simulink model "qless_forgetting_factor_16x16"  (R2021a)
settings: Solver=FixedStepDiscrete  StartTime=0.0  StopTime=stoptime*inf  RelTol=1e-3
InitFcn:
  | qless_init_16chan_fi
undefined symbols (not defined in the file): fc, numArrayElements, physconst, srcAngles, sv, Ts
libraries: hdlsllib x137, commfilt2 x4, commrfcorlib x3, commsync2 x3, commrflib2 x2, commrandsrc3 x2, phasedtxrxlib x2, commdigbbndcpm2 x1, simulink x1, embreciprocals x1, commdigbbndpm3 x1
(part 15 of 22)

== matlab function qless_forgetting_factor_16x16/MVDR_QLess_HDL/Complex Partial-Systolic Matrix Solve Using Q-less QR Decomposition with Forgetting Factor Manually Tiled n=16/Complex Partial-Systolic Q-less QR with Forgetting Factor/Complex Partial-Systolic Q-less QR with Forgetting Factor Manually tiled/Complex Partial-Systolic Q-less QR Decomposition with Forgetting Factor Section Constant pivot2/Partial-Systolic Q-less QR with Forgetting Factor Memory Controller/MATLAB Function ==
  data: xIn input; xOut output; aIn input; validIn input size=1; validRowRotationInput input size=1; restart input size=1; yOut output; processRowRotations output size=1; validOut output size=1; ready output size=1; n parameter size=1
function [...
        xOut,...
        yOut,...
        processRowRotations,...
        validOut,...
        ready...
        ] = ...
        partialSystolicQlessQRMemoryControllerForgettingFactorMATLAB(...
        xIn,...
        aIn,...
        validIn,...
        validRowRotationInput,...
        restart, ...
        n)
    
    % Persistent states
    persistent mState
    persistent mRow
    persistent mR
    
    if isempty(mState)
        mState = uint8(0);
        mRow = uint16(1);
        mR = zeros(1,n,'like',aIn);
    end
    
    [...
        xOut,...
        yOut,...
        processRowRotations,...
        validOut,...
        ready,...
        mState,...
        mRow,...
        mR...
        ] = ...
        partialSystolicQlessQRMemoryControllerForgettingFactor(...
        xIn,...
        aIn,...
        validIn,...
        validRowRotationInput,...
        restart, ...
        n,...
        mState,...
        mRow,...
        mR);
end

function [...
        xOut,...
        yOut,...
        processRowRotations,...
        validOut,...
        ready,...
        mState,...
        mRowIndex,...
        mRow...
        ] = ...
        partialSystolicQlessQRMemoryControllerForgettingFactor(...
        xIn,...
        aIn,...
        validIn,...
        validRowRotationInput,...
        restart, ...
        n,...
        mState,...
        mRowIndex,...
        mRow)
    %partialSystolicQlessQRMemoryControllerForgettingFactor
    
    % Copyright 2020 The MathWorks, Inc.
    %#codegen
    
    % State names
    NEWMATRIX = uint8(0);
    GETROW = uint8(1);
    PROCESSPIVOT = uint8(2);
    OUTPUTROW = uint8(3);
    
    % Get states
    state = mState;
    row = mRowIndex;
    
    if restart
        state = NEWMATRIX;
    end
    
    % Default outputs.  States change them as needed.
    xOut = mRow;
    yOut = aIn;
    processRowRotations = false;
    validOut = false;
    ready = false;
    
    switch state
        case NEWMATRIX
            mRow(:) = 0;
            mRowIndex(:) = 1;
            mState(:) = GETROW;
            ready(:) = true;
        case GETROW
            if  validIn
                processRowRotations = true;
                mRowIndex(:) = row + 1;
                mState(:) = PROCESSPIVOT;
            else
                ready = true;
            end
        case PROCESSPIVOT
            if validRowRotationInput
                mRow(:) = xIn;
                if row > n
                    mState(:) = OUTPUTROW;
                else
                    mState(:) = GETROW;
                end
            end
        case OUTPUTROW
            validOut = true;
            mState(:) = GETROW;
    end
end

== matlab function qless_forgetting_factor_16x16/MVDR_QLess_HDL/Complex Partial-Systolic Matrix Solve Using Q-less QR Decomposition with Forgetting Factor Manually Tiled n=16/Complex Partial-Systolic Q-less QR with Forgetting Factor/Complex Partial-Systolic Q-less QR with Forgetting Factor Manually tiled/Complex Partial-Systolic Q-less QR Decomposition with Forgetting Factor Section Constant pivot1/Complex Partial-Systolic Q-less QR Row Rotations/Q-less QR 2nd and 3rd Quadrant Compensation ==
  settings: fimath=hdlfimath
  data: x input size=[1,n]; y input size=[1,n]; xOut output size=[1,n]; yOut output size=[1,n]; pivot parameter size=1
function [xOut, yOut] = quadrantCompensation(x, y, pivot)
    %quadrantCompensation Quadrant adjustment by reflection through the origin.
    %   [XOUT, YOUT, UOUT, VOUT] = QUADRANT_COMPENSATION(X,Y,U,V,PIVOT)
    %   reflects the points (x,y) and (u,v) through the origin if (x,y)
    %   lies in the 3rd or 4th quadrant. This brings the points into the
    %   1st and 2nd quadrants for CORDIC algorithms.
    
    %   Copyright 2018 The MathWorks, Inc.
    %#codegen

   if real(x(pivot))<0
        % Compensation for 3rd and 4th quadrants
        xOut = -x;
        yOut = -y;
    else
        xOut = x;
        yOut = y;
    end


end

== matlab function qless_forgetting_factor_16x16/MVDR_QLess_HDL/Complex Partial-Systolic Matrix Solve Using Q-less QR Decomposition with Forgetting Factor Manually Tiled n=16/Complex Partial-Systolic Q-less QR with Forgetting Factor/Complex Partial-Systolic Q-less QR with Forgetting Factor Manually tiled/Complex Partial-Systolic Q-less QR Decomposition with Forgetting Factor Section Constant pivot3/Complex Partial-Systolic Q-less QR Row Rotations/Complex Partial-Systolic Q-less QR CORDIC Row Rotation/CORDIC QR Kernel ==
  settings: fimath=hdlfimath
  data: xIn input; yIn input; validIn input; restart input; xOut output size=[1 n]; yOut output size=[1 n]; n parameter; validOut output boolean; ready output; pivot parameter size=1
function [xOut, yOut, validOut, ready] = cordic_qr_row_rotation(...
                                                xIn, yIn,...
                                                validIn,...
                                                restart,...
                                                n, pivot)... 
    %CORDIC_QR_ROW_ROTATION performs one CORDIC Givens rotation
    % [XOUT, YOUT] = CORDIC_QR_ROW_ROTATION(...
    %                                       XREG,YREG,...
    %                                       XIN,YIN,...
    %                                       pivot,...
    %                                       STILLITERATING, ITERATION)
    % performs one iteration of the CORDIC Givens rotation according to
    % the formula below.
    %
    % if real(y(column)) < 0
    %       xOut = x - y/2^iteration
    %       yOut = y + x/2^iteration
    %   else
    %       xOut = x + y/2^iteration
    %       yOut = y - x/2^iteration
    % end
    %
    % The values for X, Y, are taken from XIN, YIN, on the first iteration, 
    % and XREG, YREG on succeeding iterations.
    
    %   Copyright 2018 The MathWorks, Inc.
    
    %#codegen
    
    % Initialize variables to set datatypes
    
    persistent xReg yReg count readyReg
    
    
    
    fixed.emblib.internal.cordicRowRotations.checkValidDatatypes(xIn, yIn,'x','y', 'cordic_qr_row_rotation');
    T = fixed.emblib.internal.cordicRowRotations.getTypesTable(xIn,xIn);
    maxNIters = coder.const(fixed.emblib.internal.cordicRowRotations.getMaxNIters(xIn));
    
    if isempty(xReg)
       xReg = zeros(1,n,'like',T.x);
       yReg = zeros(1,n,'like',T.y);
       count = cast(0,'like',T.count);
       readyReg = true;
    end
    
    if validIn
        iteration = cast(0,'like',count);
        x = cast(xIn,'like',T.x);
        y = cast(yIn,'like',T.y);
    else
        iteration = count;
        x = xReg;
        y = yReg;
    end
    
    [xNext, yNext] = cordicQlessQRRowRotation(x, y, iteration, pivot, T);
    incrCounter =  (validIn && readyReg) || (iteration > 0 && iteration < maxNIters);
    if restart || ~incrCounter
        iterationNext = cast(0,'like',T.count);
    else
        iterationNext = cast(iteration + 1,'like',T.count);
    end
    
    if restart || (iteration == maxNIters - 1)
        readyNext = true;
    elseif validIn && ~readyReg
        readyNext = false;
    else
        readyNext = readyReg;
    end
        
        
    % Set the output
    xOut = xNext;
    yOut = yNext;
    if iteration == maxNIters - 1
        validOut = true;
        % Set the registers to zero to prevent overflows being reported on
        % CORDIC iterations over invalid data.
        xReg(:) = 0;
        yReg(:) = 0;
    else
        validOut = false;
        % Still iterating, so update the registers with next values.    
        xReg(:) = xNext;
        yReg(:) = yNext;
    end
    ready = readyNext;
    % Update the registers
    count(:) = iterationNext;
    readyReg(:) = readyNext;
    
end

function [xOut, yOut] = cordicQlessQRRowRotation(x, y,...
        iteration, pivot, T)
%cordicQlessQRRowRotation One iteration of the Q-less QR CORDIC kernel
%   [XOUT, YOUT] = cordicQlessQRRowRotation(X,Y,...
%                                      ITERATION, PIVOT, T)
%   performs a single CORDIC Givens rotation according to the
%   formula below
%
%   if real(y(pivot)) < 0
%       xOut = x - y/2^iteration
%       yOut = y + x/2^iteration
%   else
%       xOut = x + y/2^iteration
%       yOut = y - x/2^iteration
%   end

    coder.inline('always');
    
    % Initialize output variables
    xOut = cast(x,'like',T.x);
    yOut = cast(y,'like',T.y);
    % Right shift the inputs for CORDIC rotations.
    x1 = zeros(size(x),'like',x);
    y1 = zeros(size(y),'like',y);
    coder.unroll
    for k = pivot:length(x)
        x1(k) = bitsra(x(k), iteration);
        y1(k) = bitsra(y(k), iteration);
    end
    if real(y(pivot)) < 0
        % Counter-clockwise rotation
        coder.unroll
        for k = pivot:length(x)
            xOut(k) = x(k) - y1(k);
            yOut(k) = y(k) + x1(k);
        end
    else
        % Clockwise rotation
        coder.unroll
        for k = pivot:length(x)
            xOut(k) = x(k) + y1(k);
            yOut(k) = y(k) - x1(k);
        end
    end
end

== matlab function qless_forgetting_factor_16x16/MVDR_QLess_HDL/Complex Partial-Systolic Matrix Solve Using Q-less QR Decomposition with Forgetting Factor Manually Tiled n=16/Complex Partial-Systolic Q-less QR with Forgetting Factor/Complex Partial-Systolic Q-less QR with Forgetting Factor Manually tiled/Complex Partial-Systolic Q-less QR Decomposition with Forgetting Factor Section Constant pivot3/Complex Partial-Systolic Q-less QR Row Rotations/Inverse CORDIC Gain1/MATLAB Function ==
  data: u input; y output
function y = inverseCORDICGain(u)
    %inverseCORDICGain Multiply by the inverse of the CORDIC gain constant
    %   Y = inverseCORDICGain(U) multiplies input U by the inverse CORDIC
    %   gain constant.  The data type of output Y is the same as the data
    %   type of input U.  This data type will never overflow because the
    %   inverse CORDIC gain constant quickly converges to around 0.60725 as
    %   a function of the word length of the input.
    F = fixed.fimathLike(u);
    [~, Kn] = fixed.cordicConstants(u);
    y = setfimath(u,F) * Kn;
end

== matlab function qless_forgetting_factor_16x16/MVDR_QLess_HDL/Complex Partial-Systolic Matrix Solve Using Q-less QR Decomposition with Forgetting Factor Manually Tiled n=16/Complex Partial-Systolic Q-less QR with Forgetting Factor/Complex Partial-Systolic Q-less QR with Forgetting Factor Manually tiled/Complex Partial-Systolic Q-less QR Decomposition with Forgetting Factor Section Constant pivot3/Complex Partial-Systolic Q-less QR Row Rotations/Inverse CORDIC Gain4/MATLAB Function ==
  data: u input; y output
function y = inverseCORDICGain(u)
    %inverseCORDICGain Multiply by the inverse of the CORDIC gain constant
    %   Y = inverseCORDICGain(U) multiplies input U by the inverse CORDIC
    %   gain constant.  The data type of output Y is the same as the data
    %   type of input U.  This data type will never overflow because the
    %   inverse CORDIC gain constant quickly converges to around 0.60725 as
    %   a function of the word length of the input.
    F = fixed.fimathLike(u);
    [~, Kn] = fixed.cordicConstants(u);
    y = setfimath(u,F) * Kn;
end

== matlab function qless_forgetting_factor_16x16/MVDR_QLess_HDL/Complex Partial-Systolic Matrix Solve Using Q-less QR Decomposition with Forgetting Factor Manually Tiled n=16/Complex Partial-Systolic Q-less QR with Forgetting Factor/Complex Partial-Systolic Q-less QR with Forgetting Factor Manually tiled/Complex Partial-Systolic Q-less QR Decomposition with Forgetting Factor Section Constant pivot3/Complex Partial-Systolic Q-less QR Row Rotations/Q-less QR 2nd and 3rd Quadrant Compensation ==
  settings: fimath=hdlfimath
  data: x input size=[1,n]; y input size=[1,n]; xOut output size=[1,n]; yOut output size=[1,n]; pivot parameter size=1
function [xOut, yOut] = quadrantCompensation(x, y, pivot)
    %quadrantCompensation Quadrant adjustment by reflection through the origin.
    %   [XOUT, YOUT, UOUT, VOUT] = QUADRANT_COMPENSATION(X,Y,U,V,PIVOT)
    %   reflects the points (x,y) and (u,v) through the origin if (x,y)
    %   lies in the 3rd or 4th quadrant. This brings the points into the
    %   1st and 2nd quadrants for CORDIC algorithms.
    
    %   Copyright 2018 The MathWorks, Inc.
    %#codegen

   if real(x(pivot))<0
        % Compensation for 3rd and 4th quadrants
        xOut = -x;
        yOut = -y;
    else
        xOut = x;
        yOut = y;
    end


end

== matlab function qless_forgetting_factor_16x16/MVDR_QLess_HDL/Complex Partial-Systolic Matrix Solve Using Q-less QR Decomposition with Forgetting Factor Manually Tiled n=16/Complex Partial-Systolic Q-less QR with Forgetting Factor/Complex Partial-Systolic Q-less QR with Forgetting Factor Manually tiled/Complex Partial-Systolic Q-less QR Decomposition with Forgetting Factor Section Constant pivot3/Complex Partial-Systolic Q-less QR Row Rotations/Q-less QR Rotate First Element To Real1/Q-less QR Real Row Rotations/Inverse CORDIC Gain/MATLAB Function ==
  data: u input; y output
function y = inverseCORDICGain(u)
    %inverseCORDICGain Multiply by the inverse of the CORDIC gain constant
    %   Y = inverseCORDICGain(U) multiplies input U by the inverse CORDIC
    %   gain constant.  The data type of output Y is the same as the data
    %   type of input U.  This data type will never overflow because the
    %   inverse CORDIC gain constant quickly converges to around 0.60725 as
    %   a function of the word length of the input.
    F = fixed.fimathLike(u);
    [~, Kn] = fixed.cordicConstants(u);
    y = setfimath(u,F) * Kn;
end

== matlab function qless_forgetting_factor_16x16/MVDR_QLess_HDL/Complex Partial-Systolic Matrix Solve Using Q-less QR Decomposition with Forgetting Factor Manually Tiled n=16/Complex Partial-Systolic Q-less QR with Forgetting Factor/Complex Partial-Systolic Q-less QR with Forgetting Factor Manually tiled/Complex Partial-Systolic Q-less QR Decomposition with Forgetting Factor Section Constant pivot3/Complex Partial-Systolic Q-less QR Row Rotations/Q-less QR Rotate First Element To Real1/Q-less QR Real Row Rotations/Inverse CORDIC Gain1/MATLAB Function ==
  data: u input; y output
function y = inverseCORDICGain(u)
    %inverseCORDICGain Multiply by the inverse of the CORDIC gain constant
    %   Y = inverseCORDICGain(U) multiplies input U by the inverse CORDIC
    %   gain constant.  The data type of output Y is the same as the data
    %   type of input U.  This data type will never overflow because the
    %   inverse CORDIC gain constant quickly converges to around 0.60725 as
    %   a function of the word length of the input.
    F = fixed.fimathLike(u);
    [~, Kn] = fixed.cordicConstants(u);
    y = setfimath(u,F) * Kn;
end

== matlab function qless_forgetting_factor_16x16/MVDR_QLess_HDL/Complex Partial-Systolic Matrix Solve Using Q-less QR Decomposition with Forgetting Factor Manually Tiled n=16/Complex Partial-Systolic Q-less QR with Forgetting Factor/Complex Partial-Systolic Q-less QR with Forgetting Factor Manually tiled/Complex Partial-Systolic Q-less QR Decomposition with Forgetting Factor Section Constant pivot3/Complex Partial-Systolic Q-less QR Row Rotations/Q-less QR Rotate First Element To Real1/Q-less QR Real Row Rotations/Q-less QR Real Indexed CORDIC Row Rotation/CORDIC QR Kernel ==
  settings: fimath=hdlfimath
  data: xIn input size=n; yIn input size=n; validIn input; restart input; xOut output size=n; yOut output size=n; n parameter; validOut output boolean; ready output; pivot parameter size=1
function [xOut, yOut, validOut, ready] = cordic_qr_row_rotation(...
                                                xIn, yIn,...
                                                validIn,...
                                                restart,...
                                                n, pivot)... 
    %CORDIC_QR_ROW_ROTATION performs one CORDIC Givens rotation
    % [XOUT, YOUT] = CORDIC_QR_ROW_ROTATION(...
    %                                       XREG,YREG,...
    %                                       XIN,YIN,...
    %                                       PIVOT,...
    %                                       STILLITERATING, ITERATION)
    % performs one iteration of the CORDIC Givens rotation according to
    % the formula below.
    %
    % if real(y(column)) < 0
    %       xOut = x - y/2^iteration
    %       yOut = y + x/2^iteration
    %   else
    %       xOut = x + y/2^iteration
    %       yOut = y - x/2^iteration
    % end
    %
    % The values for X, Y, are taken from XIN, YIN, on the first iteration, 
    % and XREG, YREG on succeeding iterations.
    
    %   Copyright 2018 The MathWorks, Inc.
    
    %#codegen
    
    % Initialize variables to set datatypes
    
    persistent xReg yReg count readyReg
    
    
    
    fixed.emblib.internal.cordicRowRotations.checkValidDatatypes(xIn, yIn,'x','y', 'cordic_qr_row_rotation');
    T = fixed.emblib.internal.cordicRowRotations.getTypesTable(xIn,xIn);
    maxNIters = coder.const(fixed.emblib.internal.cordicRowRotations.getMaxNIters(xIn));
    
    if isempty(xReg)
       xReg = zeros(n,1,'like',T.x);
       yReg = zeros(n,1,'like',T.y);
       count = cast(0,'like',T.count);
       readyReg = true;
    end
    
    if validIn
        iteration = cast(0,'like',count);
        x = cast(xIn,'like',T.x);
        y = cast(yIn,'like',T.y);
    else
        iteration = count;
        x = xReg;
        y = yReg;
    end
    
    
    [xNext, yNext] = cordicQlessQRRowRotation(x, y, iteration, pivot, T);
    incrCounter =  (validIn && readyReg) || (iteration > 0 && iteration < maxNIters);
    if restart || ~incrCounter
        iterationNext = cast(0,'like',T.count);
    else
        iterationNext = cast(iteration + 1,'like',T.count);
    end
    
    if restart || (iteration == maxNIters - 1)
        readyNext = true;
    elseif validIn && ~readyReg
        readyNext = false;
    else
        readyNext = readyReg;
    end
        
        
    % Set the output
    xOut = xNext;
    yOut = yNext;
    if iteration == maxNIters - 1
        validOut = true;
        % Set the registers to zero to prevent overflows being reported on
        % CORDIC iterations over invalid data.
        xReg(:) = 0;
        yReg(:) = 0;
    else
        validOut = false;
        % Still iterating, so update the registers with next values.
        xReg(:) = xNext;
        yReg(:) = yNext;
    end
    ready = readyNext;
    % Update the registers
    count(:) = iterationNext;
    readyReg(:) = readyNext;
    
    
end

function [xOut, yOut] = cordicQlessQRRowRotation(x, y,...
        iteration, pivot, T)
%cordicQlessQRRowRotation One iteration of the Q-less QR CORDIC kernel
%   [XOUT, YOUT] = cordicQlessQRRowRotation(X,Y,...
%                                      ITERATION, PIVOT, T)
%   performs a single CORDIC Givens rotation according to the
%   formula below
%
%   if real(y(pivot)) < 0
%       xOut = x - y/2^iteration
%       yOut = y + x/2^iteration
%   else
%       xOut = x + y/2^iteration
%       yOut = y - x/2^iteration
%   end

    coder.inline('always');
    
    % Initialize output variables
    xOut = cast(x,'like',T.x);
    yOut = cast(y,'like',T.y);
    % Right shift the inputs for CORDIC rotations.
    x1 = zeros(size(x),'like',x);
    y1 = zeros(size(y),'like',y);
    coder.unroll
    for k = pivot:length(x)
        x1(k) = bitsra(x(k), iteration);
        y1(k) = bitsra(y(k), iteration);
    end
    if real(y(pivot)) < 0
        % Counter-clockwise rotation
        coder.unroll
        for k = pivot:length(x)
            xOut(k) = x(k) - y1(k);
            yOut(k) = y(k) + x1(k);
        end
    else
        % Clockwise rotation
        coder.unroll
        for k = pivot:length(x)
            xOut(k) = x(k) + y1(k);
            yOut(k) = y(k) - x1(k);
        end
    end
end

== matlab function qless_forgetting_factor_16x16/MVDR_QLess_HDL/Complex Partial-Systolic Matrix Solve Using Q-less QR Decomposition with Forgetting Factor Manually Tiled n=16/Complex Partial-Systolic Q-less QR with Forgetting Factor/Complex Partial-Systolic Q-less QR with Forgetting Factor Manually tiled/Complex Partial-Systolic Q-less QR Decomposition with Forgetting Factor Section Constant pivot3/Complex Partial-Systolic Q-less QR Row Rotations/Q-less QR Rotate First Element To Real1/Q-less QR Real Row Rotations/QR 2nd and 3rd Quadrant Compensation ==
  settings: fimath=hdlfimath
  data: x input; y input; xOut output; yOut output; pivot parameter size=1
function [xOut, yOut] = quadrantCompensation(x, y, pivot)
    %quadrantCompensation Quadrant adjustment by reflection through the origin.
    %   [XOUT, YOUT, UOUT, VOUT] = QUADRANT_COMPENSATION(X,Y,U,V,PIVOT)
    %   reflects the points (x,y) and (u,v) through the origin if (x,y)
    %   lies in the 3rd or 4th quadrant. This brings the points into the
    %   1st and 2nd quadrants for CORDIC algorithms.
    
    %   Copyright 2018 The MathWorks, Inc.
    %#codegen

    if real(x(pivot))<0
        % Compensation for 3rd and 4th quadrants
        xOut = -x;
        yOut = -y;
    else
        xOut = x;
        yOut = y;
    end

end

== matlab function qless_forgetting_factor_16x16/MVDR_QLess_HDL/Complex Partial-Systolic Matrix Solve Using Q-less QR Decomposition with Forgetting Factor Manually Tiled n=16/Complex Partial-Systolic Q-less QR with Forgetting Factor/Complex Partial-Systolic Q-less QR with Forgetting Factor Manually tiled/Complex Partial-Systolic Q-less QR Decomposition with Forgetting Factor Section Constant pivot3/Complex Partial-Systolic Q-less QR Row Rotations/Q-less QR Rotate First Element To Real1/Q-less QR Real Row Rotations/Set Element To Zero/Set Element To Zero ==
  settings: fimath=hdlfimath
  data: u input size=[1 n]; y output size=[1 n]; n parameter; pivot parameter size=1
function y = set_element_equal_to_zero(u, n, pivot)
    % SET_ELEMENT_EQUAL_TO_ZERO Zeros an element for a row-vector.
    %   Y = SET_ELEMENT_EQUAL_TO_ZERO(U, PIVOT) sets an element
    %   (specified by PIVOT) of the row-vector U to zero.

    %   Copyright 2018 The MathWorks, Inc.

    %# codegen
    assert(isequal(size(u),[1,n]));
    y = u;
    if pivot > 0 && pivot <= n
        y(pivot) = 0;
    end
end

== matlab function qless_forgetting_factor_16x16/MVDR_QLess_HDL/Complex Partial-Systolic Matrix Solve Using Q-less QR Decomposition with Forgetting Factor Manually Tiled n=16/Complex Partial-Systolic Q-less QR with Forgetting Factor/Complex Partial-Systolic Q-less QR with Forgetting Factor Manually tiled/Complex Partial-Systolic Q-less QR Decomposition with Forgetting Factor Section Constant pivot3/Complex Partial-Systolic Q-less QR Row Rotations/Set Element To Zero1/Set Element To Zero ==
  settings: fimath=hdlfimath
  data: u input size=[1 n]; y output size=[1 n]; n parameter; pivot parameter size=1
function y = set_element_equal_to_zero(u, n, pivot)
    % SET_ELEMENT_EQUAL_TO_ZERO Zeros an element for a row-vector.
    %   Y = SET_ELEMENT_EQUAL_TO_ZERO(U, PIVOT) sets an element
    %   (specified by PIVOT) of the row-vector U to zero.

    %   Copyright 2018 The MathWorks, Inc.

    %# codegen
    assert(isequal(size(u),[1,n]));
    y = u;
    if pivot > 0 && pivot <= n
        y(pivot) = 0;
    end
end

== matlab function qless_forgetting_factor_16x16/MVDR_QLess_HDL/Complex Partial-Systolic Matrix Solve Using Q-less QR Decomposition with Forgetting Factor Manually Tiled n=16/Complex Partial-Systolic Q-less QR with Forgetting Factor/Complex Partial-Systolic Q-less QR with Forgetting Factor Manually tiled/Complex Partial-Systolic Q-less QR Decomposition with Forgetting Factor Section Constant pivot10/Complex Partial-Systolic Q-less QR Row Rotations/Q-less QR Rotate First Element To Real1/Q-less QR Real Row Rotations/Inverse CORDIC Gain/MATLAB Function ==
  data: u input; y output
function y = inverseCORDICGain(u)
    %inverseCORDICGain Multiply by the inverse of the CORDIC gain constant
    %   Y = inverseCORDICGain(U) multiplies input U by the inverse CORDIC
    %   gain constant.  The data type of output Y is the same as the data
    %   type of input U.  This data type will never overflow because the
    %   inverse CORDIC gain constant quickly converges to around 0.60725 as
    %   a function of the word length of the input.
    F = fixed.fimathLike(u);
    [~, Kn] = fixed.cordicConstants(u);
    y = setfimath(u,F) * Kn;
end

== matlab function qless_forgetting_factor_16x16/MVDR_QLess_HDL/Complex Partial-Systolic Matrix Solve Using Q-less QR Decomposition with Forgetting Factor Manually Tiled n=16/Complex Partial-Systolic Q-less QR with Forgetting Factor/Complex Partial-Systolic Q-less QR with Forgetting Factor Manually tiled/Complex Partial-Systolic Q-less QR Decomposition with Forgetting Factor Section Constant pivot3/Partial-Systolic Q-less QR with Forgetting Factor Memory Controller/MATLAB Function ==
  data: xIn input; xOut output; aIn input; validIn input size=1; validRowRotationInput input size=1; restart input size=1; yOut output; processRowRotations output size=1; validOut output size=1; ready output size=1; n parameter size=1
function [...
        xOut,...
        yOut,...
        processRowRotations,...
        validOut,...
        ready...
        ] = ...
        partialSystolicQlessQRMemoryControllerForgettingFactorMATLAB(...
        xIn,...
        aIn,...
        validIn,...
        validRowRotationInput,...
        restart, ...
        n)
    
    % Persistent states
    persistent mState
    persistent mRow
    persistent mR
    
    if isempty(mState)
        mState = uint8(0);
        mRow = uint16(1);
        mR = zeros(1,n,'like',aIn);
    end
    
    [...
        xOut,...
        yOut,...
        processRowRotations,...
        validOut,...
        ready,...
        mState,...
        mRow,...
        mR...
        ] = ...
        partialSystolicQlessQRMemoryControllerForgettingFactor(...
        xIn,...
        aIn,...
        validIn,...
        validRowRotationInput,...
        restart, ...
        n,...
        mState,...
        mRow,...
        mR);
end

function [...
        xOut,...
        yOut,...
        processRowRotations,...
        validOut,...
        ready,...
        mState,...
        mRowIndex,...
        mRow...
        ] = ...
        partialSystolicQlessQRMemoryControllerForgettingFactor(...
        xIn,...
        aIn,...
        validIn,...
        validRowRotationInput,...
        restart, ...
        n,...
        mState,...
        mRowIndex,...
        mRow)
    %partialSystolicQlessQRMemoryControllerForgettingFactor
    
    % Copyright 2020 The MathWorks, Inc.
    %#codegen
    
    % State names
    NEWMATRIX = uint8(0);
    GETROW = uint8(1);
    PROCESSPIVOT = uint8(2);
    OUTPUTROW = uint8(3);
    
    % Get states
    state = mState;
    row = mRowIndex;
    
    if restart
        state = NEWMATRIX;
    end
    
    % Default outputs.  States change them as needed.
    xOut = mRow;
    yOut = aIn;
    processRowRotations = false;
    validOut = false;
    ready = false;
    
    switch state
        case NEWMATRIX
            mRow(:) = 0;
            mRowIndex(:) = 1;
            mState(:) = GETROW;
            ready(:) = true;
        case GETROW
            if  validIn
                processRowRotations = true;
                mRowIndex(:) = row + 1;
                mState(:) = PROCESSPIVOT;
            else
                ready = true;
            end
        case PROCESSPIVOT
            if validRowRotationInput
                mRow(:) = xIn;
                if row > n
                    mState(:) = OUTPUTROW;
                else
                    mState(:) = GETROW;
                end
            end
        case OUTPUTROW
            validOut = true;
            mState(:) = GETROW;
    end
end

== matlab function qless_forgetting_factor_16x16/MVDR_QLess_HDL/Complex Partial-Systolic Matrix Solve Using Q-less QR Decomposition with Forgetting Factor Manually Tiled n=16/Complex Partial-Systolic Q-less QR with Forgetting Factor/Complex Partial-Systolic Q-less QR with Forgetting Factor Manually tiled/Complex Partial-Systolic Q-less QR Decomposition with Forgetting Factor Section Constant pivot4/Complex Partial-Systolic Q-less QR Row Rotations/Complex Partial-Systolic Q-less QR CORDIC Row Rotation/CORDIC QR Kernel ==
  settings: fimath=hdlfimath
  data: xIn input; yIn input; validIn input; restart input; xOut output size=[1 n]; yOut output size=[1 n]; n parameter; validOut output boolean; ready output; pivot parameter size=1
function [xOut, yOut, validOut, ready] = cordic_qr_row_rotation(...
                                                xIn, yIn,...
                                                validIn,...
                                                restart,...
                                                n, pivot)... 
    %CORDIC_QR_ROW_ROTATION performs one CORDIC Givens rotation
    % [XOUT, YOUT] = CORDIC_QR_ROW_ROTATION(...
    %                                       XREG,YREG,...
    %                                       XIN,YIN,...
    %                                       pivot,...
    %                                       STILLITERATING, ITERATION)
    % performs one iteration of the CORDIC Givens rotation according to
    % the formula below.
    %
    % if real(y(column)) < 0
    %       xOut = x - y/2^iteration
    %       yOut = y + x/2^iteration
    %   else
    %       xOut = x + y/2^iteration
    %       yOut = y - x/2^iteration
    % end
    %
    % The values for X, Y, are taken from XIN, YIN, on the first iteration, 
    % and XREG, YREG on succeeding iterations.
    
    %   Copyright 2018 The MathWorks, Inc.
    
    %#codegen
    
    % Initialize variables to set datatypes
    
    persistent xReg yReg count readyReg
    
    
    
    fixed.emblib.internal.cordicRowRotations.checkValidDatatypes(xIn, yIn,'x','y', 'cordic_qr_row_rotation');
    T = fixed.emblib.internal.cordicRowRotations.getTypesTable(xIn,xIn);
    maxNIters = coder.const(fixed.emblib.internal.cordicRowRotations.getMaxNIters(xIn));
    
    if isempty(xReg)
       xReg = zeros(1,n,'like',T.x);
       yReg = zeros(1,n,'like',T.y);
       count = cast(0,'like',T.count);
       readyReg = true;
    end
    
    if validIn
        iteration = cast(0,'like',count);
        x = cast(xIn,'like',T.x);
        y = cast(yIn,'like',T.y);
    else
        iteration = count;
        x = xReg;
        y = yReg;
    end
    
    [xNext, yNext] = cordicQlessQRRowRotation(x, y, iteration, pivot, T);
    incrCounter =  (validIn && readyReg) || (iteration > 0 && iteration < maxNIters);
    if restart || ~incrCounter
        iterationNext = cast(0,'like',T.count);
    else
        iterationNext = cast(iteration + 1,'like',T.count);
    end
    
    if restart || (iteration == maxNIters - 1)
        readyNext = true;
    elseif validIn && ~readyReg
        readyNext = false;
    else
        readyNext = readyReg;
    end
        
        
    % Set the output
    xOut = xNext;
    yOut = yNext;
    if iteration == maxNIters - 1
        validOut = true;
        % Set the registers to zero to prevent overflows being reported on
        % CORDIC iterations over invalid data.
        xReg(:) = 0;
        yReg(:) = 0;
    else
        validOut = false;
        % Still iterating, so update the registers with next values.    
        xReg(:) = xNext;
        yReg(:) = yNext;
    end
    ready = readyNext;
    % Update the registers
    count(:) = iterationNext;
    readyReg(:) = readyNext;
    
end

function [xOut, yOut] = cordicQlessQRRowRotation(x, y,...
        iteration, pivot, T)
%cordicQlessQRRowRotation One iteration of the Q-less QR CORDIC kernel
%   [XOUT, YOUT] = cordicQlessQRRowRotation(X,Y,...
%                                      ITERATION, PIVOT, T)
%   performs a single CORDIC Givens rotation according to the
%   formula below
%
%   if real(y(pivot)) < 0
%       xOut = x - y/2^iteration
%       yOut = y + x/2^iteration
%   else
%       xOut = x + y/2^iteration
%       yOut = y - x/2^iteration
%   end

    coder.inline('always');
    
    % Initialize output variables
    xOut = cast(x,'like',T.x);
    yOut = cast(y,'like',T.y);
    % Right shift the inputs for CORDIC rotations.
    x1 = zeros(size(x),'like',x);
    y1 = zeros(size(y),'like',y);
    coder.unroll
    for k = pivot:length(x)
        x1(k) = bitsra(x(k), iteration);
        y1(k) = bitsra(y(k), iteration);
    end
    if real(y(pivot)) < 0
        % Counter-clockwise rotation
        coder.unroll
        for k = pivot:length(x)
            xOut(k) = x(k) - y1(k);
            yOut(k) = y(k) + x1(k);
        end
    else
        % Clockwise rotation
        coder.unroll
        for k = pivot:length(x)
            xOut(k) = x(k) + y1(k);
            yOut(k) = y(k) - x1(k);
        end
    end
end

== matlab function qless_forgetting_factor_16x16/MVDR_QLess_HDL/Complex Partial-Systolic Matrix Solve Using Q-less QR Decomposition with Forgetting Factor Manually Tiled n=16/Complex Partial-Systolic Q-less QR with Forgetting Factor/Complex Partial-Systolic Q-less QR with Forgetting Factor Manually tiled/Complex Partial-Systolic Q-less QR Decomposition with Forgetting Factor Section Constant pivot4/Complex Partial-Systolic Q-less QR Row Rotations/Inverse CORDIC Gain1/MATLAB Function ==
  data: u input; y output
function y = inverseCORDICGain(u)
    %inverseCORDICGain Multiply by the inverse of the CORDIC gain constant
    %   Y = inverseCORDICGain(U) multiplies input U by the inverse CORDIC
    %   gain constant.  The data type of output Y is the same as the data
    %   type of input U.  This data type will never overflow because the
    %   inverse CORDIC gain constant quickly converges to around 0.60725 as
    %   a function of the word length of the input.
    F = fixed.fimathLike(u);
    [~, Kn] = fixed.cordicConstants(u);
    y = setfimath(u,F) * Kn;
end

== matlab function qless_forgetting_factor_16x16/MVDR_QLess_HDL/Complex Partial-Systolic Matrix Solve Using Q-less QR Decomposition with Forgetting Factor Manually Tiled n=16/Complex Partial-Systolic Q-less QR with Forgetting Factor/Complex Partial-Systolic Q-less QR with Forgetting Factor Manually tiled/Complex Partial-Systolic Q-less QR Decomposition with Forgetting Factor Section Constant pivot4/Complex Partial-Systolic Q-less QR Row Rotations/Inverse CORDIC Gain4/MATLAB Function ==
  data: u input; y output
function y = inverseCORDICGain(u)
    %inverseCORDICGain Multiply by the inverse of the CORDIC gain constant
    %   Y = inverseCORDICGain(U) multiplies input U by the inverse CORDIC
    %   gain constant.  The data type of output Y is the same as the data
    %   type of input U.  This data type will never overflow because the
    %   inverse CORDIC gain constant quickly converges to around 0.60725 as
    %   a function of the word length of the input.
    F = fixed.fimathLike(u);
    [~, Kn] = fixed.cordicConstants(u);
    y = setfimath(u,F) * Kn;
end

== matlab function qless_forgetting_factor_16x16/MVDR_QLess_HDL/Complex Partial-Systolic Matrix Solve Using Q-less QR Decomposition with Forgetting Factor Manually Tiled n=16/Complex Partial-Systolic Q-less QR with Forgetting Factor/Complex Partial-Systolic Q-less QR with Forgetting Factor Manually tiled/Complex Partial-Systolic Q-less QR Decomposition with Forgetting Factor Section Constant pivot4/Complex Partial-Systolic Q-less QR Row Rotations/Q-less QR 2nd and 3rd Quadrant Compensation ==
  settings: fimath=hdlfimath
  data: x input size=[1,n]; y input size=[1,n]; xOut output size=[1,n]; yOut output size=[1,n]; pivot parameter size=1
function [xOut, yOut] = quadrantCompensation(x, y, pivot)
    %quadrantCompensation Quadrant adjustment by reflection through the origin.
    %   [XOUT, YOUT, UOUT, VOUT] = QUADRANT_COMPENSATION(X,Y,U,V,PIVOT)
    %   reflects the points (x,y) and (u,v) through the origin if (x,y)
    %   lies in the 3rd or 4th quadrant. This brings the points into the
    %   1st and 2nd quadrants for CORDIC algorithms.
    
    %   Copyright 2018 The MathWorks, Inc.
    %#codegen

   if real(x(pivot))<0
        % Compensation for 3rd and 4th quadrants
        xOut = -x;
        yOut = -y;
    else
        xOut = x;
        yOut = y;
    end


end

== matlab function qless_forgetting_factor_16x16/MVDR_QLess_HDL/Complex Partial-Systolic Matrix Solve Using Q-less QR Decomposition with Forgetting Factor Manually Tiled n=16/Complex Partial-Systolic Q-less QR with Forgetting Factor/Complex Partial-Systolic Q-less QR with Forgetting Factor Manually tiled/Complex Partial-Systolic Q-less QR Decomposition with Forgetting Factor Section Constant pivot4/Complex Partial-Systolic Q-less QR Row Rotations/Q-less QR Rotate First Element To Real1/Q-less QR Real Row Rotations/Inverse CORDIC Gain/MATLAB Function ==
  data: u input; y output
function y = inverseCORDICGain(u)
    %inverseCORDICGain Multiply by the inverse of the CORDIC gain constant
    %   Y = inverseCORDICGain(U) multiplies input U by the inverse CORDIC
    %   gain constant.  The data type of output Y is the same as the data
    %   type of input U.  This data type will never overflow because the
    %   inverse CORDIC gain constant quickly converges to around 0.60725 as
    %   a function of the word length of the input.
    F = fixed.fimathLike(u);
    [~, Kn] = fixed.cordicConstants(u);
    y = setfimath(u,F) * Kn;
end

== matlab function qless_forgetting_factor_16x16/MVDR_QLess_HDL/Complex Partial-Systolic Matrix Solve Using Q-less QR Decomposition with Forgetting Factor Manually Tiled n=16/Complex Partial-Systolic Q-less QR with Forgetting Factor/Complex Partial-Systolic Q-less QR with Forgetting Factor Manually tiled/Complex Partial-Systolic Q-less QR Decomposition with Forgetting Factor Section Constant pivot10/Complex Partial-Systolic Q-less QR Row Rotations/Q-less QR Rotate First Element To Real1/Q-less QR Real Row Rotations/Inverse CORDIC Gain1/MATLAB Function ==
  data: u input; y output
function y = inverseCORDICGain(u)
    %inverseCORDICGain Multiply by the inverse of the CORDIC gain constant
    %   Y = inverseCORDICGain(U) multiplies input U by the inverse CORDIC
    %   gain constant.  The data type of output Y is the same as the data
    %   type of input U.  This data type will never overflow because the
    %   inverse CORDIC gain constant quickly converges to around 0.60725 as
    %   a function of the word length of the input.
    F = fixed.fimathLike(u);
    [~, Kn] = fixed.cordicConstants(u);
    y = setfimath(u,F) * Kn;
end

== matlab function qless_forgetting_factor_16x16/MVDR_QLess_HDL/Complex Partial-Systolic Matrix Solve Using Q-less QR Decomposition with Forgetting Factor Manually Tiled n=16/Complex Partial-Systolic Q-less QR with Forgetting Factor/Complex Partial-Systolic Q-less QR with Forgetting Factor Manually tiled/Complex Partial-Systolic Q-less QR Decomposition with Forgetting Factor Section Constant pivot4/Complex Partial-Systolic Q-less QR Row Rotations/Q-less QR Rotate First Element To Real1/Q-less QR Real Row Rotations/Inverse CORDIC Gain1/MATLAB Function ==
  data: u input; y output
function y = inverseCORDICGain(u)
    %inverseCORDICGain Multiply by the inverse of the CORDIC gain constant
    %   Y = inverseCORDICGain(U) multiplies input U by the inverse CORDIC
    %   gain constant.  The data type of output Y is the same as the data
    %   type of input U.  This data type will never overflow because the
    %   inverse CORDIC gain constant quickly converges to around 0.60725 as
    %   a function of the word length of the input.
    F = fixed.fimathLike(u);
    [~, Kn] = fixed.cordicConstants(u);
    y = setfimath(u,F) * Kn;
end

== matlab function qless_forgetting_factor_16x16/MVDR_QLess_HDL/Complex Partial-Systolic Matrix Solve Using Q-less QR Decomposition with Forgetting Factor Manually Tiled n=16/Complex Partial-Systolic Q-less QR with Forgetting Factor/Complex Partial-Systolic Q-less QR with Forgetting Factor Manually tiled/Complex Partial-Systolic Q-less QR Decomposition with Forgetting Factor Section Constant pivot4/Complex Partial-Systolic Q-less QR Row Rotations/Q-less QR Rotate First Element To Real1/Q-less QR Real Row Rotations/Q-less QR Real Indexed CORDIC Row Rotation/CORDIC QR Kernel ==
  settings: fimath=hdlfimath
  data: xIn input size=n; yIn input size=n; validIn input; restart input; xOut output size=n; yOut output size=n; n parameter; validOut output boolean; ready output; pivot parameter size=1
function [xOut, yOut, validOut, ready] = cordic_qr_row_rotation(...
                                                xIn, yIn,...
                                                validIn,...
                                                restart,...
                                                n, pivot)... 
    %CORDIC_QR_ROW_ROTATION performs one CORDIC Givens rotation
    % [XOUT, YOUT] = CORDIC_QR_ROW_ROTATION(...
    %                                       XREG,YREG,...
    %                                       XIN,YIN,...
    %                                       PIVOT,...
    %                                       STILLITERATING, ITERATION)
    % performs one iteration of the CORDIC Givens rotation according to
    % the formula below.
    %
    % if real(y(column)) < 0
    %       xOut = x - y/2^iteration
    %       yOut = y + x/2^iteration
    %   else
    %       xOut = x + y/2^iteration
    %       yOut = y - x/2^iteration
    % end
    %
    % The values for X, Y, are taken from XIN, YIN, on the first iteration, 
    % and XREG, YREG on succeeding iterations.
    
    %   Copyright 2018 The MathWorks, Inc.
    
    %#codegen
    
    % Initialize variables to set datatypes
    
    persistent xReg yReg count readyReg
    
    
    
    fixed.emblib.internal.cordicRowRotations.checkValidDatatypes(xIn, yIn,'x','y', 'cordic_qr_row_rotation');
    T = fixed.emblib.internal.cordicRowRotations.getTypesTable(xIn,xIn);
    maxNIters = coder.const(fixed.emblib.internal.cordicRowRotations.getMaxNIters(xIn));
    
    if isempty(xReg)
       xReg = zeros(n,1,'like',T.x);
       yReg = zeros(n,1,'like',T.y);
       count = cast(0,'like',T.count);
       readyReg = true;
    end
    
    if validIn
        iteration = cast(0,'like',count);
        x = cast(xIn,'like',T.x);
        y = cast(yIn,'like',T.y);
    else
        iteration = count;
        x = xReg;
        y = yReg;
    end
    
    
    [xNext, yNext] = cordicQlessQRRowRotation(x, y, iteration, pivot, T);
    incrCounter =  (validIn && readyReg) || (iteration > 0 && iteration < maxNIters);
    if restart || ~incrCounter
        iterationNext = cast(0,'like',T.count);
    else
        iterationNext = cast(iteration + 1,'like',T.count);
    end
    
    if restart || (iteration == maxNIters - 1)
        readyNext = true;
    elseif validIn && ~readyReg
        readyNext = false;
    else
        readyNext = readyReg;
    end
        
        
    % Set the output
    xOut = xNext;
    yOut = yNext;
    if iteration == maxNIters - 1
        validOut = true;
        % Set the registers to zero to prevent overflows being reported on
        % CORDIC iterations over invalid data.
        xReg(:) = 0;
        yReg(:) = 0;
    else
        validOut = false;
        % Still iterating, so update the registers with next values.
        xReg(:) = xNext;
        yReg(:) = yNext;
    end
    ready = readyNext;
    % Update the registers
    count(:) = iterationNext;
    readyReg(:) = readyNext;
    
    
end

function [xOut, yOut] = cordicQlessQRRowRotation(x, y,...
        iteration, pivot, T)
%cordicQlessQRRowRotation One iteration of the Q-less QR CORDIC kernel
%   [XOUT, YOUT] = cordicQlessQRRowRotation(X,Y,...
%                                      ITERATION, PIVOT, T)
%   performs a single CORDIC Givens rotation according to the
%   formula below
%
%   if real(y(pivot)) < 0
%       xOut = x - y/2^iteration
%       yOut = y + x/2^iteration
%   else
%       xOut = x + y/2^iteration
%       yOut = y - x/2^iteration
%   end

    coder.inline('always');
    
    % Initialize output variables
    xOut = cast(x,'like',T.x);
    yOut = cast(y,'like',T.y);
    % Right shift the inputs for CORDIC rotations.
    x1 = zeros(size(x),'like',x);
    y1 = zeros(size(y),'like',y);
    coder.unroll
    for k = pivot:length(x)
        x1(k) = bitsra(x(k), iteration);
        y1(k) = bitsra(y(k), iteration);
    end
    if real(y(pivot)) < 0
        % Counter-clockwise rotation
        coder.unroll
        for k = pivot:length(x)
            xOut(k) = x(k) - y1(k);
            yOut(k) = y(k) + x1(k);
        end
    else
        % Clockwise rotation
        coder.unroll
        for k = pivot:length(x)
            xOut(k) = x(k) + y1(k);
            yOut(k) = y(k) - x1(k);
        end
    end
end

== matlab function qless_forgetting_factor_16x16/MVDR_QLess_HDL/Complex Partial-Systolic Matrix Solve Using Q-less QR Decomposition with Forgetting Factor Manually Tiled n=16/Complex Partial-Systolic Q-less QR with Forgetting Factor/Complex Partial-Systolic Q-less QR with Forgetting Factor Manually tiled/Complex Partial-Systolic Q-less QR Decomposition with Forgetting Factor Section Constant pivot4/Complex Partial-Systolic Q-less QR Row Rotations/Q-less QR Rotate First Element To Real1/Q-less QR Real Row Rotations/QR 2nd and 3rd Quadrant Compensation ==
  settings: fimath=hdlfimath
  data: x input; y input; xOut output; yOut output; pivot parameter size=1
function [xOut, yOut] = quadrantCompensation(x, y, pivot)
    %quadrantCompensation Quadrant adjustment by reflection through the origin.
    %   [XOUT, YOUT, UOUT, VOUT] = QUADRANT_COMPENSATION(X,Y,U,V,PIVOT)
    %   reflects the points (x,y) and (u,v) through the origin if (x,y)
    %   lies in the 3rd or 4th quadrant. This brings the points into the
    %   1st and 2nd quadrants for CORDIC algorithms.
    
    %   Copyright 2018 The MathWorks, Inc.
    %#codegen

    if real(x(pivot))<0
        % Compensation for 3rd and 4th quadrants
        xOut = -x;
        yOut = -y;
    else
        xOut = x;
        yOut = y;
    end

end

== matlab function qless_forgetting_factor_16x16/MVDR_QLess_HDL/Complex Partial-Systolic Matrix Solve Using Q-less QR Decomposition with Forgetting Factor Manually Tiled n=16/Complex Partial-Systolic Q-less QR with Forgetting Factor/Complex Partial-Systolic Q-less QR with Forgetting Factor Manually tiled/Complex Partial-Systolic Q-less QR Decomposition with Forgetting Factor Section Constant pivot4/Complex Partial-Systolic Q-less QR Row Rotations/Q-less QR Rotate First Element To Real1/Q-less QR Real Row Rotations/Set Element To Zero/Set Element To Zero ==
  settings: fimath=hdlfimath
  data: u input size=[1 n]; y output size=[1 n]; n parameter; pivot parameter size=1
function y = set_element_equal_to_zero(u, n, pivot)
    % SET_ELEMENT_EQUAL_TO_ZERO Zeros an element for a row-vector.
    %   Y = SET_ELEMENT_EQUAL_TO_ZERO(U, PIVOT) sets an element
    %   (specified by PIVOT) of the row-vector U to zero.

    %   Copyright 2018 The MathWorks, Inc.

    %# codegen
    assert(isequal(size(u),[1,n]));
    y = u;
    if pivot > 0 && pivot <= n
        y(pivot) = 0;
    end
end

== matlab function qless_forgetting_factor_16x16/MVDR_QLess_HDL/Complex Partial-Systolic Matrix Solve Using Q-less QR Decomposition with Forgetting Factor Manually Tiled n=16/Complex Partial-Systolic Q-less QR with Forgetting Factor/Complex Partial-Systolic Q-less QR with Forgetting Factor Manually tiled/Complex Partial-Systolic Q-less QR Decomposition with Forgetting Factor Section Constant pivot4/Complex Partial-Systolic Q-less QR Row Rotations/Set Element To Zero1/Set Element To Zero ==
  settings: fimath=hdlfimath
  data: u input size=[1 n]; y output size=[1 n]; n parameter; pivot parameter size=1
function y = set_element_equal_to_zero(u, n, pivot)
    % SET_ELEMENT_EQUAL_TO_ZERO Zeros an element for a row-vector.
    %   Y = SET_ELEMENT_EQUAL_TO_ZERO(U, PIVOT) sets an element
    %   (specified by PIVOT) of the row-vector U to zero.

    %   Copyright 2018 The MathWorks, Inc.

    %# codegen
    assert(isequal(size(u),[1,n]));
    y = u;
    if pivot > 0 && pivot <= n
        y(pivot) = 0;
    end
end
